simulink model "StaticSynchronousSeriesCompensator"  (R2024a)
settings: Solver=ode23tb  StartTime=0  StopTime=10  MaxStep=1/60  RelTol=1e-4  AbsTol=1e-3
undefined symbols (not defined in the file or in its folder): D1, Delta
libraries: spsPower3phPhasorLib x5, spsThreePhaseVIMeasurementLib x4, spsDistributedParametersLineLib x4, spsSequenceAnalyzerPhasorLib x4, spsThreePhaseParallelRLCLoadLib x3, spsSynchronousMachinepuStandardLib x2, spsThreePhaseTransformerTwoWindingsLib x2, spsStairGeneratorLib x2, spsFirstOrderFilterLib x2, spsExcitationSystemLib x2, spsGenericPowerSystemStabilizerLib x2, spsHydraulicTurbineandGovernorLib x2
settings Model: Creator=The MathWorks, Inc.  LastModifiedBy=Monia
settings SolverCC: AutoScaleAbsTol=off  AlgebraicLoopSolver=TrustRegion
settings DataIOCC: SaveFinalState=on  SaveFormat=Array  SaveOutput=off  SaveTime=off  ReturnWorkspaceOutputs=off  SignalLoggingName=sigsOut
settings OptimizationCC: BooleanDataType=off  ExpressionDepthLimit=2147483647  InitFltsAndDblsToZero=on  LifeSpan=inf
settings DebuggingCC: UnderspecifiedInitializationDetection=Classic  MergeDetectMultiDrivingBlocksExec=none  CheckExecutionContextPreStartOutputMsg=on  SignalResolutionControl=TryResolveAllWithWarning  MultiTaskDSMMsg=warning  MultiTaskCondExecSysMsg=none  SigSpecEnsureSampleTimeMsg=none  FcnCallInpInsideContextMsg=warning  UnconnectedInputMsg=warning  UnconnectedOutputMsg=warning  StateNameClashWarn=warning  SFUnexpectedBacktrackingDiag=warning  SFNoUnconditionalDefaultTransitionDiag=warning  SFExecutionAtInitializationDiag=none  ArithmeticOperatorsInVariantConditions=warning
settings HardwareCC: ProdBitPerPointer=32  ProdBitPerSizeT=32  ProdBitPerPtrDiffT=32  ProdLargestAtomicFloat=None  ProdIntDivRoundTo=Undefined  ProdEndianess=Unspecified  ProdWordSize=32  ProdHWDeviceType=32-bit Generic  TargetUnknown=on
settings ModelReferenceCC: EnableRefExpFcnMdlSchedulingChecks=on  PropagateSignalLabelsOutOfModel=off
settings SFSimCC: SimUseLocalCustomCode=off  CustomCodeUndefinedFunction=UseInterfaceOnly
settings RTWCC: RTWUseLocalCustomCode=off  GPUComputeCapability=3.5  DLArmComputeVersion=19.05
settings CodeAppCC: StateflowObjectComments=on
settings GRTTargetCC: TargetLangStandard=C89/C90 (ANSI)  CombineOutputUpdateFcns=off  GRTInterface=on
settings ConfigComp: CovMetricSettings=dw  CovSaveCumulativeToWorkspaceVar=on  CovSaveSingleToWorkspaceVar=on  CovExternalEMLEnable=off  CovSFcnEnable=off
settings SimscapeCC: SimscapeNormalizeSystem=off

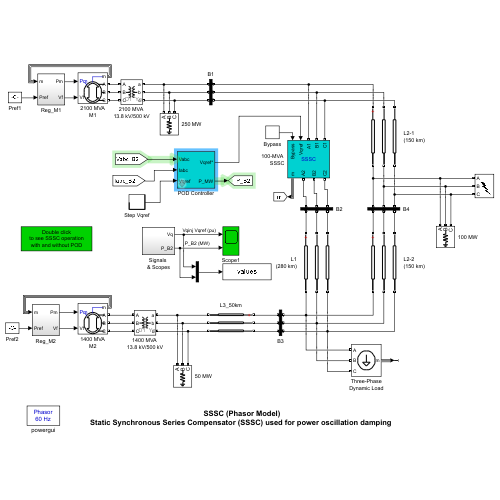
[thumbnail: Simulink's stored preview of the top-level diagram]
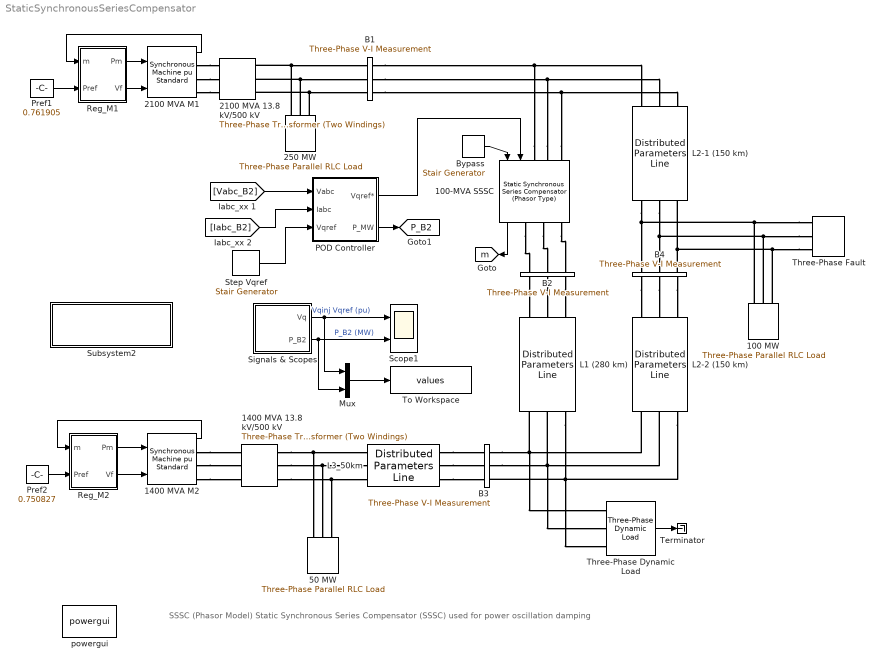
== system StaticSynchronousSeriesCompensator ==
  note: SSSC (Phasor Model)
      | Static Synchronous Series Compensator (SSSC) used for power oscillation damping
  100 MW : spsThreePhaseParallelRLCLoadLib/Three-Phase Parallel RLC Load  LConnTagsString=A|B|C  Configuration=Y (grounded)  NominalVoltage=500e3  Vabc=[1e3 1e3 1e3]  Vabcp=[1e3 1e3 1e3]  NominalFrequency=60  UnbalancedPower=off  ActivePower=100e6  InductivePower=0  CapacitivePower=0  Pabc=[10e3 9e3 11e3]  QLabc=[100 90 110]  QCabc=[100 90 110]  Pabcp=[10e3 9e3 11e3]  QLabcp=[100 90 110]  QCabcp=[100 90 110]  Measurements=None  LoadType=constant Z
  100-MVA SSSC : factslib/Power-Electronics Based FACTS/Static Synchronous Series Compensator (Phasor Type)  SystemNominal=[ 500e3, 60 ]  SeriesNominal=[ 100e6, 0.1]  RL=[ 0.16/30, 0.16 ]  Iinit=[ 0 0]  VnomDC=40000  C_DC=375e-6  ExternalByPass=External control  Vqref=0.05  ExternalVqref=on  MaxRateVqRef=0.5  Par_VacReg=[0.03 1.5]/8  Par_VdcReg=[0.1e-3 20e-3]
  1400 MVA M2 : spsSynchronousMachinepuStandardLib/Synchronous Machine pu Standard  PresetModel=No  MechanicalLoad=Mechanical power Pm  ShowDetailedParameters=on  RotorType=Salient-pole  Units=per unit standard parameters  MeasurementBus=off  NominalParameters="[1400E6  13800   60 ]"  Reactances1=[ 31 32 33 34 35 36 37 ]  Reactances2=[ 1.305, 0.296, 0.252, 0.474, 0.243, 0.18 ]  dAxisTimeConstants=Short-circuit  qAxisTimeConstants=Open-circuit  TimeConstants1=[]  TimeConstants2=[]  TimeConstants3=[]  TimeConstants4=[]  TimeConstants5=[ 1.01, 0.053, 0.1 ]  TimeConstants6=[]  TimeConstants7=[]  TimeConstants8=[]  StatorResistance=2.8544e-3  Mechanical="[ 3.7 0  32]"  PolePairs=32  InitialConditions=[0 -71.2244 0.745111 0.745111 0.745111 -3.89206 -123.892 116.108 1.33295]  SetSaturation=off  Saturation=[0.6404,0.7127,0.8441,0.9214,0.9956,1.082,1.19,1.316,1.457;0.7,0.7698,0.8872,0.9466,0.9969,1.046,1.1,1.151,1.201]  LoadFlowParameters=[2 1000000000 13938 0 0]  TsPowergui=0  TsBlock=-1  IterativeModel=Forward Euler  IterativeDiscreteModel=Trapezoidal non iterative  BusType=PV  Pref=0  Qref=0  Qmin=-inf  Qmax=inf  PLF=0  QLF=0
  1400 MVA 13.8 kV/500 kV : spsThreePhaseTransformerTwoWindingsLib/Three-Phase Transformer (Two Windings)  Winding1Connection=Delta (D1)  Winding2Connection=Yg  CoreType=Three single-phase transformers  SetSaturation=off  Hysteresis=off  DataFile='basic_model'  SetInitialFlux=off  Measurements=None  UNITS=pu  NominalPower=[ 1400e6 60 ]  Winding1="[ 13.8e3 0.002  0.0]"  Winding2=[ 500e3 0.002 0.12]  Rm=500  Lm=500  L0=0.5  Saturation="[ 0,0  ;  0.005,1.2  ;  1.0,1.4 ]"  InitialFluxes=[ 0.8 , -0.8 , 0.7 ]  BreakLoop=off  DiscreteSolver=Trapezoidal iterative  DataType=off  TransfoNumber=0
  2100 MVA M1 : spsSynchronousMachinepuStandardLib/Synchronous Machine pu Standard  PresetModel=No  MechanicalLoad=Mechanical power Pm  ShowDetailedParameters=on  RotorType=Salient-pole  Units=per unit standard parameters  MeasurementBus=off  NominalParameters="[2100E6  13800   60 ]"  Reactances1=[ 31 32 33 34 35 36 37 ]  Reactances2=[ 1.305, 0.296, 0.252, 0.474, 0.243, 0.18 ]  dAxisTimeConstants=Short-circuit  qAxisTimeConstants=Open-circuit  TimeConstants1=[]  TimeConstants2=[]  TimeConstants3=[]  TimeConstants4=[]  TimeConstants5=[ 1.01, 0.053, 0.1 ]  TimeConstants6=[]  TimeConstants7=[]  TimeConstants8=[]  StatorResistance=2.8544e-3  Mechanical="[ 3.7 0  32]"  PolePairs=32  InitialConditions=[0 -58.9841 0.763417 0.763417 0.763417 14.3746 -105.625 134.375 1.2256]  SetSaturation=off  Saturation=[0.6404,0.7127,0.8441,0.9214,0.9956,1.082,1.19,1.316,1.457;0.7,0.7698,0.8872,0.9466,0.9969,1.046,1.1,1.151,1.201]  LoadFlowParameters=[1 1600000000 0 0 0]  TsPowergui=0  TsBlock=-1  IterativeModel=Forward Euler  IterativeDiscreteModel=Trapezoidal non iterative  BusType=PV  Pref=0  Qref=0  Qmin=-inf  Qmax=inf  PLF=0  QLF=0
  2100 MVA 13.8 kV/500 kV : spsThreePhaseTransformerTwoWindingsLib/Three-Phase Transformer (Two Windings)  Winding1Connection=Delta (D1)  Winding2Connection=Yg  CoreType=Three single-phase transformers  SetSaturation=off  Hysteresis=off  DataFile='basic_model'  SetInitialFlux=off  Measurements=None  UNITS=pu  NominalPower=[ 2100e6 60 ]  Winding1="[ 13.8e3 0.002  0.0]"  Winding2=[ 500e3 0.002 0.12]  Rm=500  Lm=500  L0=0.5  Saturation="[ 0,0  ;  0.005,1.2  ;  1.0,1.4 ]"  InitialFluxes=[ 0.8 , -0.8 , 0.7 ]  BreakLoop=off  DiscreteSolver=Trapezoidal iterative  DataType=off  TransfoNumber=0
  250 MW : spsThreePhaseParallelRLCLoadLib/Three-Phase Parallel RLC Load  LConnTagsString=A|B|C  Configuration=Y (grounded)  NominalVoltage=500e3  Vabc=[1e3 1e3 1e3]  Vabcp=[1e3 1e3 1e3]  NominalFrequency=60  UnbalancedPower=off  ActivePower=250e6  InductivePower=0  CapacitivePower=0  Pabc=[10e3 9e3 11e3]  QLabc=[100 90 110]  QCabc=[100 90 110]  Pabcp=[10e3 9e3 11e3]  QLabcp=[100 90 110]  QCabcp=[100 90 110]  Measurements=None  LoadType=constant Z
  50 MW : spsThreePhaseParallelRLCLoadLib/Three-Phase Parallel RLC Load  LConnTagsString=A|B|C  Configuration=Y (grounded)  NominalVoltage=500e3  Vabc=[1e3 1e3 1e3]  Vabcp=[1e3 1e3 1e3]  NominalFrequency=60  UnbalancedPower=off  ActivePower=50e6  InductivePower=0  CapacitivePower=0  Pabc=[10e3 9e3 11e3]  QLabc=[100 90 110]  QCabc=[100 90 110]  Pabcp=[10e3 9e3 11e3]  QLabcp=[100 90 110]  QCabcp=[100 90 110]  Measurements=None  LoadType=constant Z
  B1 : spsThreePhaseVIMeasurementLib/Three-Phase V-I Measurement  VoltageMeasurement=phase-to-ground  SetLabelV=on  LabelV=Vabc_B1  Vpu=on  VpuLL=off  CurrentMeasurement=yes  SetLabelI=on  LabelI=Iabc_B1  Ipu=on  Pbase=100e6  Vbase=500e3  OutputType=Complex  PhasorSimulation=on  PSBequivalent=0
  B2 : spsThreePhaseVIMeasurementLib/Three-Phase V-I Measurement  VoltageMeasurement=phase-to-ground  SetLabelV=on  LabelV=Vabc_B2  Vpu=on  VpuLL=off  CurrentMeasurement=yes  SetLabelI=on  LabelI=Iabc_B2  Ipu=on  Pbase=100e6  Vbase=500e3  OutputType=Complex  PhasorSimulation=on  PSBequivalent=0
  B3 : spsThreePhaseVIMeasurementLib/Three-Phase V-I Measurement  VoltageMeasurement=phase-to-ground  SetLabelV=on  LabelV=Vabc_B3  Vpu=on  VpuLL=off  CurrentMeasurement=yes  SetLabelI=on  LabelI=Iabc_B3  Ipu=on  Pbase=100e6  Vbase=500e3  OutputType=Complex  PhasorSimulation=on  PSBequivalent=0
  B4 : spsThreePhaseVIMeasurementLib/Three-Phase V-I Measurement  VoltageMeasurement=phase-to-ground  SetLabelV=on  LabelV=Vabc_B4  Vpu=on  VpuLL=off  CurrentMeasurement=yes  SetLabelI=on  LabelI=Iabc_B4  Ipu=on  Pbase=100e6  Vbase=500e3  OutputType=Complex  PhasorSimulation=on  PSBequivalent=0
  Bypass : spsStairGeneratorLib/Stair Generator  t=[0, 0.1]  e=[1, 0 ]  Ts=0
  L1 (280 km) : spsDistributedParametersLineLib/Distributed Parameters Line  Phases=3  Length=280  Frequency=60  Resistance=[0.01273*2 0.3864]  Inductance="[0.9337e-3  4.1264e-3]"  Capacitance=[12.74e-9 7.751e-9]  x1=[2.02010775288888e-08 503561.742499164 503558.494191362;376.991118430775 376.991118430775 376.991118430775;0.458609957840964 0.780216052862194 -0.790594575681271]  x2=[1.84432192957555e-08 501044.608029119 501043.044254851;376.991118430775 376.991118430775 376.991118430775;1.52155125485832 0.525215697960913 -1.04559729553157]  x3=[5.86231045525403e-11 574.048887013091 574.037523203622;376.991118430775 376.991118430775 376.991118430775;0.876888416315659 0.35321089782295 -1.21763359755104]  x4=[2.02156349007769e-11 3100.04743027775 3100.04312365634;376.991118430775 376.991118430775 376.991118430775;-1.73681895340481 0.491334265820617 -1.07947217838417]  x5=0.00158351638758808  V1=ones(3,3)  V2=ones(3,3)  I1=ones(3,3)  I2=ones(3,3)  nHarmo=1  Measurements=None  Decoupling=off  VsMag0=0  VrMag0=0  VsAngle0=0  VrAngle0=0  IsMag0=0  IrMag0=0  IsAngle0=0  IrAngle0=0
      settings: AttributesFormatString=\n
  L2-1 (150 km) : spsDistributedParametersLineLib/Distributed Parameters Line  Phases=3  Length=150  Frequency=60  Resistance=[0.01273*2 0.3864]  Inductance="[0.9337e-3  4.1264e-3]"  Capacitance=[12.74e-9 7.751e-9]  x1=[1.00351256643384e-08 503561.874348524 503558.626041409;376.991118430775 376.991118430775 376.991118430775;1.71074668305783 0.949245739900236 -0.621564888640289]  x2=[1.75147579524679e-08 507426.874684524 507424.367147325;376.991118430775 376.991118430775 376.991118430775;1.68304971137804 0.809960291170216 -0.760851730258501]  x3=[3.6939473436014e-11 573.013687959086 573.003252391458;376.991118430775 376.991118430775 376.991118430775;0.664012931777572 0.485888149150613 -1.08495473042395]  x4=[2.99498076794821e-11 3160.06406930413 3160.05880347047;376.991118430775 376.991118430775 376.991118430775;2.6974314372518 0.834320289689431 -0.73648649420357]  x5=0.000848312350493614  V1=ones(3,3)  V2=ones(3,3)  I1=ones(3,3)  I2=ones(3,3)  nHarmo=1  Measurements=None  Decoupling=off  VsMag0=0  VrMag0=0  VsAngle0=0  VrAngle0=0  IsMag0=0  IrMag0=0  IsAngle0=0  IrAngle0=0
      settings: AttributesFormatString=\n
  L2-2 (150 km) : spsDistributedParametersLineLib/Distributed Parameters Line  Phases=3  Length=150  Frequency=60  Resistance=[0.01273*2 0.3864]  Inductance="[0.9337e-3  4.1264e-3]"  Capacitance=[12.74e-9 7.751e-9]  x1=[1.75147579524679e-08 507426.874684524 507424.367147325;376.991118430775 376.991118430775 376.991118430775;1.68304971137804 0.809960291170216 -0.760851730258501]  x2=[1.84432192957555e-08 501044.608029119 501043.044254851;376.991118430775 376.991118430775 376.991118430775;1.79871664707738 0.69424533716147 -0.876567656331016]  x3=[3.23612806926644e-11 756.151995635004 756.140076872001;376.991118430775 376.991118430775 376.991118430775;1.55619118273107 0.707989924805799 -0.862845535514267]  x4=[1.41029178057703e-11 2942.57588529396 2942.57158696918;376.991118430775 376.991118430775 376.991118430775;1.64876095366768 0.640895650345567 -0.929910833128882]  x5=0.000848312350493614  V1=ones(3,3)  V2=ones(3,3)  I1=ones(3,3)  I2=ones(3,3)  nHarmo=1  Measurements=None  Decoupling=off  VsMag0=0  VrMag0=0  VsAngle0=0  VrAngle0=0  IsMag0=0  IrMag0=0  IsAngle0=0  IrAngle0=0
      settings: AttributesFormatString=\n
  L3_50km : spsDistributedParametersLineLib/Distributed Parameters Line  Phases=3  Length=50  Frequency=60  Resistance=[0.01273*2 0.3864]  Inductance="[0.9337e-3  4.1264e-3]"  Capacitance=[12.74e-9 7.751e-9]  x1=[1.84432192957555e-08 501044.608029119 501043.044254851;376.991118430775 376.991118430775 376.991118430775;2.0119207949382 0.824268136546514 -0.746544856945973]  x2=[2.13238941544407e-08 502570.320993889 502568.185573869;376.991118430775 376.991118430775 376.991118430775;2.02872521160294 0.893766737091725 -0.677045919938461]  x3=[5.12797770421175e-11 3815.50430371981 3815.49789928637;376.991118430775 376.991118430775 376.991118430775;1.2436268754791 0.841212242957262 -0.72959209800696]  x4=[3.50331250436798e-11 133.527393702521 133.547103354183;376.991118430775 376.991118430775 376.991118430775;-3.11510091027285 -1.88202912532793 2.83054197137128]  x5=0.000282770783497871  V1=ones(3,3)  V2=ones(3,3)  I1=ones(3,3)  I2=ones(3,3)  nHarmo=1  Measurements=None  Decoupling=off  VsMag0=0  VrMag0=0  VsAngle0=0  VrAngle0=0  IsMag0=0  IrMag0=0  IsAngle0=0  IrAngle0=0
      settings: AttributesFormatString=\n
  Mux : Mux  Inputs=2
  POD Controller : Subsystem  mask(POD Controller){podstatus=On, Kpod=0.08, Tlowpass=100e-3, Twashout=1, Tleadlag=[ 1 0.1 ], Vlimits=[ -0.1 0.1 ], Vinit=6.64}
      mask prompts: podstatus "POD status"; Kpod "Gain:"; Tlowpass "Lowpass time constant (s)"; Twashout "Wash-out time constant (s)"; Tleadlag "Lead-lag time constants: [ Tnum Tden ]"; Vlimits "Output limits (pu): [ min  max  ]"; Vinit "Initial input:"
      mask TypeOptions podstatus: Off | On
      mask Callback podstatus:
      | %
      | BlockName=[gcs,'/',get_param(gcb,'Name')];
      | if strcmp('Off',get_param(BlockName,'podstatus'));
      | 	p{2}='off';p{3}='off';p{4}='off';p{5}='off';p{6}='off';p{7}='off';
      | else
      | 	p{2}='on';p{3}='on';p{4}='on';p{5}='on';p{6}='on';p{7}='on';
      | end
      | ParVisible={'on',p{2},p{3},p{4},p{5},p{6},p{7}};
      | set_param(BlockName,'MaskVisibilities',ParVisible);
      | %
  Pref1 : Constant  Value=0.761905
  Pref2 : Constant  Value=0.750827
  Reg_M1 : Subsystem
  Reg_M2 : Subsystem
  Scope1 : Scope  NumInputPorts=2
  Signals & Scopes : Subsystem
  Step Vqref : spsStairGeneratorLib/Stair Generator  t=[ 0 2 6]*1000  e=[0.0 -0.08 0.08 ]  Ts=0
  Subsystem2 : Subsystem
      settings: OpenFcn=open('StaticSynchronousSeriesCompensator.fig')
      mask Display: disp('Double click\nto see SSSC operation\nwith and without POD')
  Terminator : Terminator
  Three-Phase Dynamic Load : spsThreePhaseDynamicLoadLib/Three-Phase Dynamic Load  NominalVoltage=[ 500e3 60 ]  ActiveReactivePowers=[2.2e+009 1e+008]  PositiveSequence=[1.00208 20.9514]  ExternalControl=off  NpNq=[1.3 2]  TimeConstants="[0  0  0  0]"  MinimumVoltage=0.7  Tfilter=1e-4  LoadFlowParameters=[4 2200000000 0 0 100000000]
  Three-Phase Fault : spsThreePhaseFaultLib/Three-Phase Fault  InitialStates=0  FaultA=on  FaultB=on  FaultC=on  GroundFault=on  SwitchTimes=[ 20/60 30/60]+1  External=off  SwitchStatus=NaN  FaultResistance=0.001  GroundResistance=0.001  SnubberResistance=1e6  SnubberCapacitance=inf  Measurements=None
  To Workspace : ToWorkspace  VariableName=values  SaveFormat=Timeseries  SampleTime=-1
  powergui : spspowerguiLib/powergui  Priority=2  SimulationMode=Phasor  SampleTime=0  frequency=60  Iterations=50  frequencyindice=60  Pbase=100e6  ErrMax=1e-4  UnitsV=kV  UnitsW=MW  buscounter=0  FunctionMessages=off  echomessages=off  EnableUseOfTLC=off  CurrentSourceSwitches=off  DisableSnubberDevices=off  DisableRonSwitches=off  DisableVfSwitches=off  DisplayEquations=off  AutomaticDiscreteSolvers=off  SolverType=Tustin  Interpol=off  ExternalGateDelay=off  methode=off  Ts=0  x0status=blocks  SPID=off  SwTol=0  HookPort=off  NonlinearTolerance=1e-4  nMaxIteration=100  ContinueOnMaxIteration=off  RestoreLinks=warning  ResistiveCurrentMeasurement=off  Frange=[0:2:500]  Ylog=off  Xlog=on  ShowGrid=off  save=off  variable=ZData  structure=0  ZoomFFT=on  StartTime=0.0  cycles=1  DisplayStyle=1  fundamental=60  FreqAxis=off  MaxFrequency=1000  frequencyindicesteady=1  RmsSteady=1  display=off
  tag scope: P_B2=global, m=global
  wires:
  Reg_M1/1(Pm) -> 2100 MVA M1/1
  Reg_M1/2(Vf) -> 2100 MVA M1/2
  Pref1/1 -> Reg_M1/2(Pref)
  2100 MVA M1/1 -> Reg_M1/1(m)
  Reg_M2/1(Pm) -> 1400 MVA M2/1
  Reg_M2/2(Vf) -> 1400 MVA M2/2
  Pref2/1 -> Reg_M2/2(Pref)
  1400 MVA M2/1 -> Reg_M2/1(m)
  100-MVA SSSC/1 -> [m]
  POD Controller/1(Vqref*) -> 100-MVA SSSC/2
  Bypass/1 -> 100-MVA SSSC/1
  POD Controller/2(P_MW) -> [P_B2]
  [Vabc_B2] -> POD Controller/1(Vabc)
  [Iabc_B2] -> POD Controller/2(Iabc)
  Three-Phase Dynamic Load/1 -> Terminator/1
  Signals & Scopes/1(Vq) -> Mux/1, Scope1/1  "Vqinj Vqref (pu)"
  Signals & Scopes/2(P_B2) -> Mux/2, Scope1/2  "P_B2 (MW)"
  Step Vqref/1 -> POD Controller/3(Vqref)
  Mux/1 -> To Workspace/1
  connections:
  2100 MVA M1/RConn1 -- 2100 MVA 13.8 kV/500 kV/LConn1
  2100 MVA M1/RConn2 -- 2100 MVA 13.8 kV/500 kV/LConn2
  2100 MVA M1/RConn3 -- 2100 MVA 13.8 kV/500 kV/LConn3
  250 MW/LConn1 -- 2100 MVA 13.8 kV/500 kV/RConn1 -- B1/LConn1
  250 MW/LConn2 -- 2100 MVA 13.8 kV/500 kV/RConn2 -- B1/LConn2
  250 MW/LConn3 -- 2100 MVA 13.8 kV/500 kV/RConn3 -- B1/LConn3
  100-MVA SSSC/LConn1 -- L2-1 (150 km)/LConn1 -- B1/RConn1
  100-MVA SSSC/LConn2 -- L2-1 (150 km)/LConn2 -- B1/RConn2
  100-MVA SSSC/LConn3 -- L2-1 (150 km)/LConn3 -- B1/RConn3
  1400 MVA M2/RConn1 -- 1400 MVA 13.8 kV/500 kV/LConn1
  1400 MVA M2/RConn2 -- 1400 MVA 13.8 kV/500 kV/LConn2
  1400 MVA M2/RConn3 -- 1400 MVA 13.8 kV/500 kV/LConn3
  B3/RConn1 -- Three-Phase Dynamic Load/LConn1 -- L2-2 (150 km)/RConn1 -- L1 (280 km)/RConn1
  B3/RConn2 -- Three-Phase Dynamic Load/LConn2 -- L2-2 (150 km)/RConn2 -- L1 (280 km)/RConn2
  B3/RConn3 -- Three-Phase Dynamic Load/LConn3 -- L1 (280 km)/RConn3 -- L2-2 (150 km)/RConn3
  B4/RConn1 -- L2-2 (150 km)/LConn1
  B4/RConn2 -- L2-2 (150 km)/LConn2
  B4/RConn3 -- L2-2 (150 km)/LConn3
  Three-Phase Fault/LConn1 -- 100 MW/LConn1 -- B4/LConn1 -- L2-1 (150 km)/RConn1
  Three-Phase Fault/LConn2 -- 100 MW/LConn2 -- B4/LConn2 -- L2-1 (150 km)/RConn2
  Three-Phase Fault/LConn3 -- 100 MW/LConn3 -- B4/LConn3 -- L2-1 (150 km)/RConn3
  1400 MVA 13.8 kV/500 kV/RConn1 -- L3_50km/RConn1 -- 50 MW/LConn1
  1400 MVA 13.8 kV/500 kV/RConn2 -- L3_50km/RConn2 -- 50 MW/LConn2
  1400 MVA 13.8 kV/500 kV/RConn3 -- L3_50km/RConn3 -- 50 MW/LConn3
  100-MVA SSSC/RConn1 -- B2/LConn1
  100-MVA SSSC/RConn2 -- B2/LConn2
  100-MVA SSSC/RConn3 -- B2/LConn3
  B2/RConn1 -- L1 (280 km)/LConn1
  B2/RConn2 -- L1 (280 km)/LConn2
  B2/RConn3 -- L1 (280 km)/LConn3
  L3_50km/LConn1 -- B3/LConn1
  L3_50km/LConn2 -- B3/LConn2
  L3_50km/LConn3 -- B3/LConn3

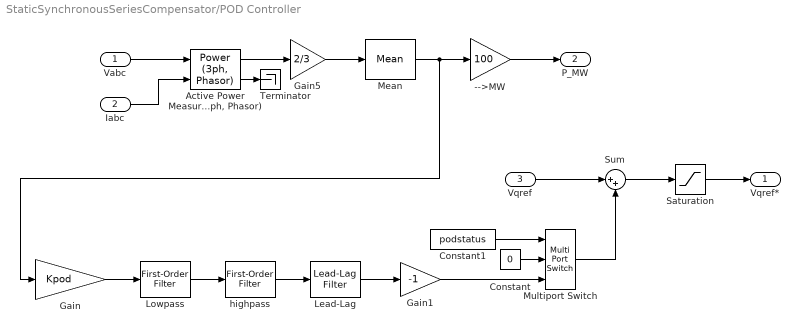
== system StaticSynchronousSeriesCompensator/POD Controller ==
  Vabc : Inport
  Iabc : Inport  Port=2
  Vqref : Inport  Port=3
  -->MW : Gain  Gain=100  SaturateOnIntegerOverflow=on  OutDataTypeStr=Inherit: Same as input  ParamDataTypeStr=Inherit: Same as input
  "Active Power Measurement (3ph, Phasor)" : spsPower3phPhasorLib/Power (3ph, Phasor)
  Constant : Constant  Value=0
  Constant1 : Constant  Value=podstatus
  Gain : Gain  Gain=Kpod
  Gain1 : Gain  Gain=-1
  Gain5 : Gain  Gain=2/3  SaturateOnIntegerOverflow=on  OutDataTypeStr=Inherit: Same as input  ParamDataTypeStr=Inherit: Same as input
  "Lead-Lag " : spsLeadLagFilterLib/Lead-Lag Filter  T1=Tleadlag(1)  T2=Tleadlag(2)  Vdc_Init=0  Ts=0
  Lowpass : spsFirstOrderFilterLib/First-Order Filter  FilterType=Lowpass  Tc=Tlowpass  Ts=0  Initialize=on  Vac_Init=[0.8 -25 60]  Vdc_Init=Vinit*Kpod  PlotResponse=off  FreqRange="[0,  200,  1]"
  Mean : spsMeanLib/Mean  Freq=60  Vinit=Vinit  Ts=0
  Multiport Switch : MultiPortSwitch  Inputs=2  SampleTime=0  SaturateOnIntegerOverflow=off  InputSameDT=off
  Saturation : Saturate  UpperLimit=Vlimits(2)  LowerLimit=Vlimits(1)
  Sum : Sum  Inputs=|++
  Terminator : Terminator
  highpass : spsFirstOrderFilterLib/First-Order Filter  FilterType=Highpass  Tc=Twashout  Ts=0  Initialize=on  Vac_Init=[0.0 -25 60]  Vdc_Init=Vinit*Kpod  PlotResponse=off  FreqRange="[0,  200,  1]"
  Vqref* : Outport  VectorParamsAs1DForOutWhenUnconnected=off
  P_MW : Outport  Port=2  VectorParamsAs1DForOutWhenUnconnected=off
  wires:
  Gain/1 -> Lowpass/1
  Vqref/1 -> Sum/1
  Sum/1 -> Saturation/1
  Saturation/1 -> Vqref*/1
  Vabc/1 -> "Active Power Measurement (3ph, Phasor)"/1
  Iabc/1 -> "Active Power Measurement (3ph, Phasor)"/2
  Lowpass/1 -> highpass/1
  Multiport Switch/1 -> Sum/2
  Constant1/1 -> Multiport Switch/1
  Constant/1 -> Multiport Switch/2
  Gain1/1 -> Multiport Switch/3
  -->MW/1 -> P_MW/1
  "Active Power Measurement (3ph, Phasor)"/1 -> Gain5/1
  "Active Power Measurement (3ph, Phasor)"/2 -> Terminator/1
  Gain5/1 -> Mean/1
  Mean/1 -> Gain/1, -->MW/1
  highpass/1 -> "Lead-Lag "/1
  "Lead-Lag "/1 -> Gain1/1

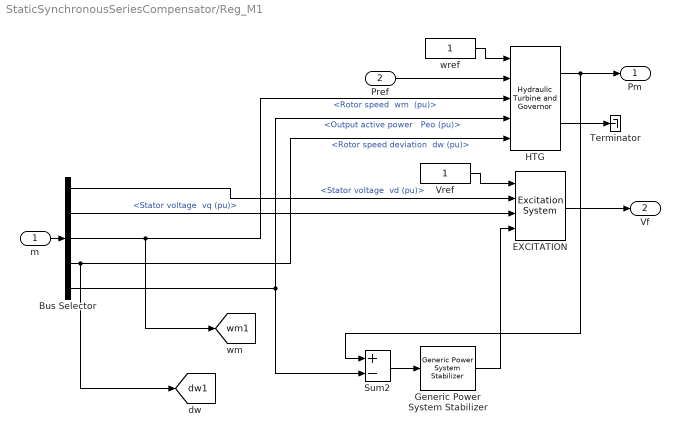
== system StaticSynchronousSeriesCompensator/Reg_M1 ==
  m : Inport
  Pref : Inport  Port=2
  Bus Selector : BusSelector  OutputSignals="dq0 components.Stator voltage  vd (pu),dq0 components.Stator voltage  vq (pu),Mechanical.Rotor speed  wm  (pu),Mechanical.Rotor speed deviation  dw (pu),Output active power   Peo (pu)"
  EXCITATION : spsExcitationSystemLib/Excitation System  tr=20e-3  reg=[ 200, 0.001 ]  exc=[ 1, 0 ]  tgr=[ 0, 0 ]  damp=[ 0.001, 0.1 ]  sat=[ 0, 0 ]  lim="[ 0,  7, 0 ]"  v0=[1,1.2256]
  Generic Power System Stabilizer : spsGenericPowerSystemStabilizerLib/Generic Power System Stabilizer  Tsensor=15e-3  K=2.5/10  Twashout=1  Tleadlag1="[0.06  1]"  Tleadlag2="[0  0]"  VSlimits=[-0.15 0.15]  Vinit=0  Plot_On=off  MagdB_On=on  FreqRange=logspace(-2,2,500)
  HTG : spsHydraulicTurbineandGovernorLib/Hydraulic Turbine and Governor  sm="[ 10/3  0.07 ]"  gate="[  0.01  0.97518  -0.1  0.1 ]"  reg="[  0.05  1.163  0.105  0  0.01  ]"  hyd="[  0  2.67  ]"  dref=0  po=0.763568
  Sum2 : Sum  Inputs=+-  InputSameDT=on  SaturateOnIntegerOverflow=on  OutDataTypeStr=Inherit: Same as first input
  Terminator : Terminator
  Vref : Constant
  wref : Constant
  Pm : Outport  InitialOutput=0  VectorParamsAs1DForOutWhenUnconnected=off
  Vf : Outport  Port=2  InitialOutput=0  VectorParamsAs1DForOutWhenUnconnected=off
  tag scope: dw1=global, wm1=global
  wires:
  Sum2/1 -> Generic Power System Stabilizer/1
  Bus Selector/1 -> EXCITATION/2  "<Stator voltage  vd (pu)>"
  EXCITATION/1 -> Vf/1
  Bus Selector/2 -> EXCITATION/3  "<Stator voltage  vq (pu)>"
  HTG/1 -> Sum2/1, Pm/1
  wref/1 -> HTG/1
  Pref/1 -> HTG/2
  Bus Selector/3 -> [wm1], HTG/3  "<Rotor speed  wm  (pu)>"
  Bus Selector/5 -> Sum2/2, HTG/4  "<Output active power   Peo (pu)>"
  Bus Selector/4 -> [dw1], HTG/5  "<Rotor speed deviation  dw (pu)>"
  m/1 -> Bus Selector/1
  Vref/1 -> EXCITATION/1
  HTG/2 -> Terminator/1
  Generic Power System Stabilizer/1 -> EXCITATION/4

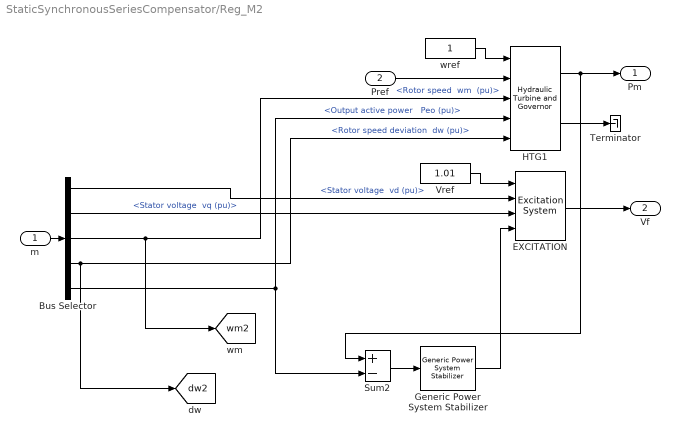
== system StaticSynchronousSeriesCompensator/Reg_M2 ==
  m : Inport
  Pref : Inport  Port=2
  Bus Selector : BusSelector  OutputSignals="dq0 components.Stator voltage  vd (pu),dq0 components.Stator voltage  vq (pu),Mechanical.Rotor speed  wm  (pu),Mechanical.Rotor speed deviation  dw (pu),Output active power   Peo (pu)"
  EXCITATION : spsExcitationSystemLib/Excitation System  tr=20e-3  reg=[ 200, 0.001 ]  exc=[ 1, 0 ]  tgr=[ 0, 0 ]  damp=[ 0.001, 0.1 ]  sat=[ 0, 0 ]  lim="[ 0,  7, 0 ]"  v0=[1.01,1.33295]
  Generic Power System Stabilizer : spsGenericPowerSystemStabilizerLib/Generic Power System Stabilizer  Tsensor=15e-3  K=2.5/10  Twashout=1  Tleadlag1="[0.06  1]"  Tleadlag2="[0  0]"  VSlimits=[-0.15 0.15]  Vinit=0  Plot_On=off  MagdB_On=on  FreqRange=logspace(-2,2,500)
  HTG1 : spsHydraulicTurbineandGovernorLib/Hydraulic Turbine and Governor  sm="[ 10/3  0.07 ]"  gate="[  0.01  0.97518  -0.1  0.1 ]"  reg="[  0.05  1.163  0.105  0  0.01  ]"  hyd="[  0  2.67  ]"  dref=0  po=0.752412
  Sum2 : Sum  Inputs=+-  InputSameDT=on  SaturateOnIntegerOverflow=on  OutDataTypeStr=Inherit: Same as first input
  Terminator : Terminator
  Vref : Constant  Value=1.01
  wref : Constant
  Pm : Outport  InitialOutput=0  VectorParamsAs1DForOutWhenUnconnected=off
  Vf : Outport  Port=2  InitialOutput=0  VectorParamsAs1DForOutWhenUnconnected=off
  tag scope: dw2=global, wm2=global
  wires:
  HTG1/2 -> Terminator/1
  Vref/1 -> EXCITATION/1
  m/1 -> Bus Selector/1
  Bus Selector/4 -> [dw2], HTG1/5  "<Rotor speed deviation  dw (pu)>"
  Bus Selector/5 -> Sum2/2, HTG1/4  "<Output active power   Peo (pu)>"
  Bus Selector/3 -> [wm2], HTG1/3  "<Rotor speed  wm  (pu)>"
  Pref/1 -> HTG1/2
  wref/1 -> HTG1/1
  HTG1/1 -> Pm/1, Sum2/1
  Bus Selector/2 -> EXCITATION/3  "<Stator voltage  vq (pu)>"
  EXCITATION/1 -> Vf/1
  Bus Selector/1 -> EXCITATION/2  "<Stator voltage  vd (pu)>"
  Sum2/1 -> Generic Power System Stabilizer/1
  Generic Power System Stabilizer/1 -> EXCITATION/4

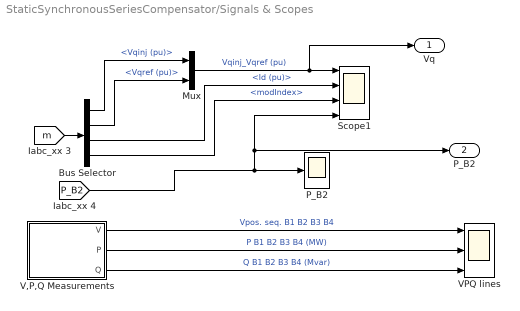
== system StaticSynchronousSeriesCompensator/Signals & Scopes ==
  Bus Selector : BusSelector  OutputSignals=Control.Vqinj (pu),Control.Vqref (pu),Control.Id (pu),Control.modIndex
  Mux : Mux  Inputs=2
  "P_B2 " : Scope
  Scope1 : Scope  NumInputPorts=4
  V,P,Q Measurements : Subsystem
      mask Display: disp('V P Q\nMeasurements')
  VPQ lines : Scope  NumInputPorts=3
  Vq : Outport  VectorParamsAs1DForOutWhenUnconnected=off
  P_B2 : Outport  Port=2  VectorParamsAs1DForOutWhenUnconnected=off
  wires:
  V,P,Q Measurements/1(V) -> VPQ lines/1  "Vpos. seq. B1 B2 B3 B4"
  V,P,Q Measurements/3(Q) -> VPQ lines/3  "Q B1 B2 B3 B4 (Mvar)"
  V,P,Q Measurements/2(P) -> VPQ lines/2  "P B1 B2 B3 B4 (MW)"
  [m] -> Bus Selector/1
  Bus Selector/1 -> Mux/1  "<Vqinj (pu)>"
  Bus Selector/2 -> Mux/2  "<Vqref (pu)>"
  Mux/1 -> Scope1/1, Vq/1  "Vqinj_Vqref (pu)"
  Bus Selector/3 -> Scope1/2  "<Id (pu)>"
  Bus Selector/4 -> Scope1/3  "<modIndex>"
  [P_B2] -> "P_B2 "/1, Scope1/4, P_B2/1

== system StaticSynchronousSeriesCompensator/Subsystem2 ==

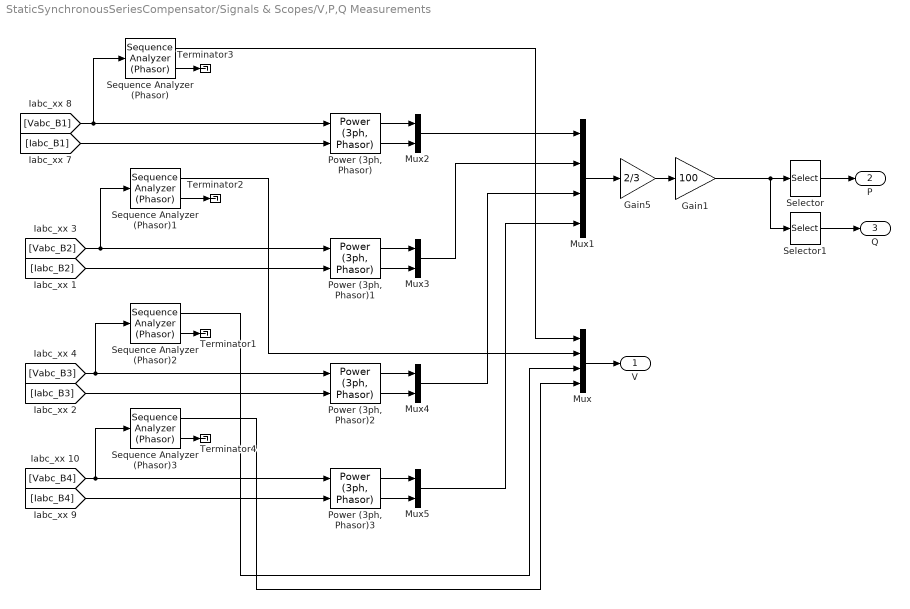
== system StaticSynchronousSeriesCompensator/Signals & Scopes/V,P,Q Measurements ==
  Gain1 : Gain  Gain=100  SaturateOnIntegerOverflow=on  OutDataTypeStr=Inherit: Same as input  ParamDataTypeStr=Inherit: Same as input
  Gain5 : Gain  Gain=2/3  SaturateOnIntegerOverflow=on  OutDataTypeStr=Inherit: Same as input  ParamDataTypeStr=Inherit: Same as input
  Mux : Mux
  Mux1 : Mux
  Mux{2..5} (4 alike) : Mux  Inputs=2
  Power (3ph, Phasor){,1..3} (4 alike) : spsPower3phPhasorLib/Power (3ph, Phasor)
  Selector : Selector  InputPortWidth=8  IndexOptions=Index vector (dialog)  Indices=[1 3 5 7 ]  OutputSizes=1
  Selector1 : Selector  InputPortWidth=8  IndexOptions=Index vector (dialog)  Indices=[1 3 5 7 ]+1  OutputSizes=1
  Sequence Analyzer (Phasor){,1..3} (4 alike) : spsSequenceAnalyzerPhasorLib/Sequence Analyzer (Phasor)  seq=Positive
  Terminator{1..4} (4 alike) : Terminator
  V : Outport  VectorParamsAs1DForOutWhenUnconnected=off
  P : Outport  Port=2  VectorParamsAs1DForOutWhenUnconnected=off
  Q : Outport  Port=3  VectorParamsAs1DForOutWhenUnconnected=off
  wires:
  Gain1/1 -> Selector/1, Selector1/1
  Gain5/1 -> Gain1/1
  Sequence Analyzer (Phasor)1/2 -> Terminator2/1
  [Vabc_B2] -> "Power (3ph, Phasor)1"/1, Sequence Analyzer (Phasor)1/1
  [Iabc_B2] -> "Power (3ph, Phasor)1"/2
  [Vabc_B3] -> "Power (3ph, Phasor)2"/1, Sequence Analyzer (Phasor)2/1
  [Iabc_B3] -> "Power (3ph, Phasor)2"/2
  Sequence Analyzer (Phasor)2/2 -> Terminator1/1
  Sequence Analyzer (Phasor)1/1 -> Mux/2
  Sequence Analyzer (Phasor)2/1 -> Mux/3
  Mux/1 -> V/1
  Mux1/1 -> Gain5/1
  Selector/1 -> P/1
  Selector1/1 -> Q/1
  Sequence Analyzer (Phasor)3/2 -> Terminator4/1
  Sequence Analyzer (Phasor)3/1 -> Mux/4
  Sequence Analyzer (Phasor)/1 -> Mux/1
  [Vabc_B1] -> "Power (3ph, Phasor)"/1, Sequence Analyzer (Phasor)/1
  [Iabc_B1] -> "Power (3ph, Phasor)"/2
  "Power (3ph, Phasor)"/2 -> Mux2/2
  "Power (3ph, Phasor)"/1 -> Mux2/1
  Mux2/1 -> Mux1/1
  Mux3/1 -> Mux1/2
  "Power (3ph, Phasor)1"/1 -> Mux3/1
  "Power (3ph, Phasor)1"/2 -> Mux3/2
  "Power (3ph, Phasor)2"/1 -> Mux4/1
  "Power (3ph, Phasor)2"/2 -> Mux4/2
  Mux4/1 -> Mux1/3
  [Vabc_B4] -> "Power (3ph, Phasor)3"/1, Sequence Analyzer (Phasor)3/1
  [Iabc_B4] -> "Power (3ph, Phasor)3"/2
  "Power (3ph, Phasor)3"/1 -> Mux5/1
  "Power (3ph, Phasor)3"/2 -> Mux5/2
  Mux5/1 -> Mux1/4
  Sequence Analyzer (Phasor)/2 -> Terminator3/1
